simulink model "gm_quad_enc_fpga_pcie_slrt"  (R2020b)
settings: Solver=FixedStepDiscrete  StartTime=0.0  StopTime=5  FixedStep=1e-3  RelTol=1e-3
PostLoadFcn:
  | try
  | cell = struct2cell(dir(fullfile(speedgoatroot_hdlb, 'hdlsrc', 'quadrature', '*.vhd')));
  | addSourceFiles = strjoin(fullfile(cell(2,:),cell(1,:)), ';');
  | hdlset_param('quadrature_example_hdlc/DUT Quadrature', 'IPCoreAdditionalFiles', addSourceFiles);
  | end
undefined symbols (not defined in the file): IO334
libraries: speedgoatlib_hdlCoder_IO3xx x8, quadrature_cpulib x1
settings Model: ModifiedByFormat=Speedgoat GmbH  Creator=Speedgoat GmbH  LastModifiedBy=Speedgoat GmbH
settings SolverCC: ConcurrentTasks=on  PositivePriorityOrder=on
settings DataIOCC: ReturnWorkspaceOutputs=off
settings OptimizationCC: BlockReduction=off  ConditionallyExecuteInputs=off  DefaultParameterBehavior=Inlined  OptimizeBlockIOStorage=off
settings DebuggingCC: AlgebraicLoopMsg=error  TasksWithSamePriorityMsg=none  ParameterOverflowMsg=warning  PregeneratedLibrarySubsystemCodeDiagnostic=none  ArithmeticOperatorsInVariantConditions=warning
settings HardwareCC: ProdBitPerLong=64  ProdLongLongMode=on  ProdHWDeviceType=Intel->x86-64 (Linux 64)  TargetBitPerPointer=64  TargetBitPerSizeT=64  TargetBitPerPtrDiffT=64  TargetLongLongMode=on  TargetIntDivRoundTo=Zero  TargetEndianess=LittleEndian  TargetWordSize=64  TargetHWDeviceType=Custom Processor->MATLAB Host Computer
settings SFSimCC: SimUseLocalCustomCode=off  CustomCodeUndefinedFunction=UseInterfaceOnly
settings RTWCC: Description=Simulink Real-Time  SystemTargetFile=slrealtime.tlc  TemplateMakefile=slrealtime_default_tmf  RTWUseLocalCustomCode=off  Toolchain=Simulink Real-Time Toolchain  BuildConfiguration=Faster Runs  CodeExecutionProfiling=on  TargetLang=C++

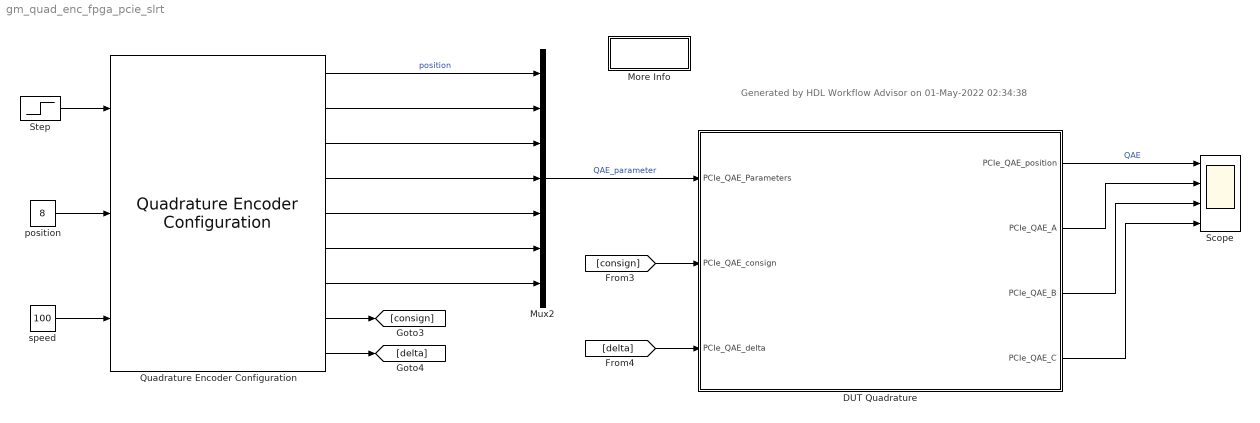
== system gm_quad_enc_fpga_pcie_slrt ==
  note: Generated by HDL Workflow Advisor on 01-May-2022 02:34:38
  DUT Quadrature : Subsystem  mask(Speedgoat IO334-325k Interface Block){module_id=1, slot=-1, ts=-1, FpgaFreq=100}
      mask prompts: module_id "FPGA Module Identifier:"; slot "PCI slot (-1: autosearch):"; ts "Sample time:"; FpgaFreq "FPGA Frequency [MHz]"
      mask help: Simulink Real-Time Interface Block for Speedgoat IO334-325k.
      mask init:
      | hdlslrt.backend.mfpgaparameters;
      mask Help: eval('speedgoatdoc_hdlc')
      mask Display:
      | SetupBlkPath = find_system(gcb, 'LookUnderMasks', 'all', 'FollowLinks', 'on', 'regexp', 'on', 'Name', 'IO3(\d|x){2}\s+Setup' );
      | SetupBlkPath = SetupBlkPath{1};
      | TS = get_param(SetupBlkPath,'timestamp_mcs');
      | disp(sprintf('Speedgoat IO334-325k\nFPGA I/O Module\n\nTimestamp\n%s\n\nReference Design\nVersion 2.1\n\nMatlab R2020b\n\nPCIe Link Width: X4\nRear Plugin: -21\nAurora Mode: None\nAurora Byteswap: true\n', TS))
  More Info : Subsystem
      settings: OpenFcn=|
      | try
      | speedgoat.hdlioblockset.doc('page', 'quadrature');
      | catch
      | web('https://www.speedgoat.com/help/hdlcoder/page/hdlb/refentry_hdl_blockset_quadrature');
      | end
      mask Display: disp('Documentation')
  Mux2 : Mux  Inputs=7
  Quadrature Encoder Configuration : quadrature_cpulib/Quadrature Encoder Configuration  fpgaFreq=100e6  n_channels=1  numSeg=[16]  phaseAngle=90  initPos=[0]  freeWheel=on
      settings: SourceProductName=Simulink Real-Time: Speedgoat HDL Blockset
  Scope : Scope  NumInputPorts=4
  Step : Step  Time=0.002
  position : Constant  Value=8  SampleTime=-1
  speed : Constant  Value=100  SampleTime=-1
  wires:
  Step/1 -> Quadrature Encoder Configuration/1
  DUT Quadrature/1(PCIe_QAE_position) -> Scope/1  "QAE"
  DUT Quadrature/4(PCIe_QAE_C) -> Scope/4
  DUT Quadrature/3(PCIe_QAE_B) -> Scope/3
  DUT Quadrature/2(PCIe_QAE_A) -> Scope/2
  Quadrature Encoder Configuration/5 -> Mux2/5
  [delta] -> DUT Quadrature/3(PCIe_QAE_delta)
  [consign] -> DUT Quadrature/2(PCIe_QAE_consign)
  Quadrature Encoder Configuration/4 -> Mux2/4
  Quadrature Encoder Configuration/1 -> Mux2/1  "position"
  Mux2/1 -> DUT Quadrature/1(PCIe_QAE_Parameters)  "QAE_parameter"
  Quadrature Encoder Configuration/9 -> [delta]
  Quadrature Encoder Configuration/8 -> [consign]
  Quadrature Encoder Configuration/7 -> Mux2/7
  Quadrature Encoder Configuration/6 -> Mux2/6
  Quadrature Encoder Configuration/3 -> Mux2/3
  Quadrature Encoder Configuration/2 -> Mux2/2
  speed/1 -> Quadrature Encoder Configuration/3
  position/1 -> Quadrature Encoder Configuration/2

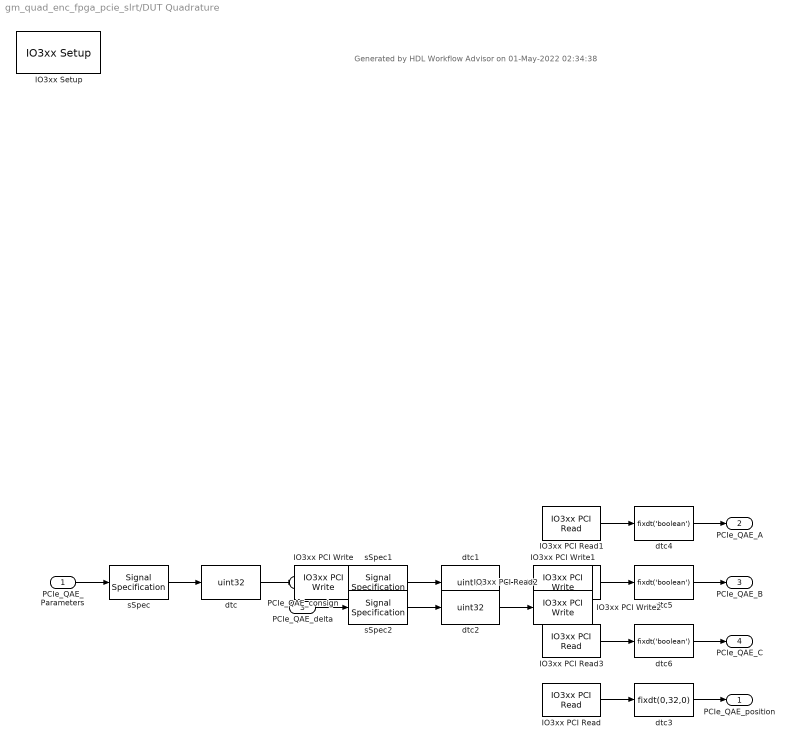
== system gm_quad_enc_fpga_pcie_slrt/DUT Quadrature ==
  note: Generated by HDL Workflow Advisor on 01-May-2022 02:34:38
  PCIe_QAE_Parameters : Inport
  PCIe_QAE_consign : Inport  Port=2  OutDataTypeStr=uint32  PortDimensions=1
  PCIe_QAE_delta : Inport  Port=3  PortDimensions=1
  IO3xx PCI Read : speedgoatlib_hdlCoder_IO3xx/IO3xx PCI Read  device_id=deviceIdx  module_id=module_id  board_type=IO3xx  port_name=PCIe_QAE_position  port_offset=hex2dec('130')  port_type=uint32  port_dim=1  strobe=0  sample_time=ts
  IO3xx PCI Read1 : speedgoatlib_hdlCoder_IO3xx/IO3xx PCI Read  device_id=deviceIdx  module_id=module_id  board_type=IO3xx  port_name=PCIe_QAE_A  port_offset=hex2dec('100')  port_type=uint32  port_dim=1  strobe=0  sample_time=ts
  IO3xx PCI Read2 : speedgoatlib_hdlCoder_IO3xx/IO3xx PCI Read  device_id=deviceIdx  module_id=module_id  board_type=IO3xx  port_name=PCIe_QAE_B  port_offset=hex2dec('104')  port_type=uint32  port_dim=1  strobe=0  sample_time=ts
  IO3xx PCI Read3 : speedgoatlib_hdlCoder_IO3xx/IO3xx PCI Read  device_id=deviceIdx  module_id=module_id  board_type=IO3xx  port_name=PCIe_QAE_C  port_offset=hex2dec('108')  port_type=uint32  port_dim=1  strobe=0  sample_time=ts
  IO3xx PCI Write : speedgoatlib_hdlCoder_IO3xx/IO3xx PCI Write  device_id=deviceIdx  module_id=module_id  board_type=IO3xx  port_name=PCIe_QAE_Parameters  port_offset=hex2dec('140')  port_type=uint32  port_dim=7  strobe=hex2dec('160')  sample_time=ts
  IO3xx PCI Write1 : speedgoatlib_hdlCoder_IO3xx/IO3xx PCI Write  device_id=deviceIdx  module_id=module_id  board_type=IO3xx  port_name=PCIe_QAE_consign  port_offset=hex2dec('128')  port_type=uint32  port_dim=1  strobe=0  sample_time=ts
  IO3xx PCI Write2 : speedgoatlib_hdlCoder_IO3xx/IO3xx PCI Write  device_id=deviceIdx  module_id=module_id  board_type=IO3xx  port_name=PCIe_QAE_delta  port_offset=hex2dec('12C')  port_type=uint32  port_dim=1  strobe=0  sample_time=ts
  IO3xx Setup : speedgoatlib_hdlCoder_IO3xx/IO3xx Setup  mdl_ss_name=quad_enc_fpga_pcie/DUT Quadrature  board_type=IO334-325k  fpga_sync_mode=on  reset_mode=on  device_id=deviceIdx  module_id=module_id  pci_slot=slot  fpga_mat_file=hdl_prj\hdlsrc\quad_enc_fpga_pcie\DUTQuadrature.mat  timestamp_mcs=05/01/22 02:23:06  timestamp=2205010147  tsreg=hex2dec('8')  bsf_file=DUTQuadrature_2205010147.mcs  mcs=0
  dtc : DataTypeConversion  OutDataTypeStr=uint32  ConvertRealWorld=Stored Integer (SI)  RndMeth=Zero
  dtc1 : DataTypeConversion  OutDataTypeStr=uint32  ConvertRealWorld=Stored Integer (SI)  RndMeth=Zero
  dtc2 : DataTypeConversion  OutDataTypeStr=uint32  ConvertRealWorld=Stored Integer (SI)  RndMeth=Zero
  dtc3 : DataTypeConversion  OutDataTypeStr=fixdt(0,32,0)  ConvertRealWorld=Stored Integer (SI)  RndMeth=Zero
  dtc4 : DataTypeConversion  OutDataTypeStr=fixdt('boolean')  ConvertRealWorld=Stored Integer (SI)  RndMeth=Zero
  dtc5 : DataTypeConversion  OutDataTypeStr=fixdt('boolean')  ConvertRealWorld=Stored Integer (SI)  RndMeth=Zero
  dtc6 : DataTypeConversion  OutDataTypeStr=fixdt('boolean')  ConvertRealWorld=Stored Integer (SI)  RndMeth=Zero
  sSpec : SignalSpecification  OutDataTypeStr=fixdt(0,32,0)
  sSpec1 : SignalSpecification  OutDataTypeStr=fixdt(0,32,0)
  sSpec2 : SignalSpecification  OutDataTypeStr=fixdt(1,32,0)
  PCIe_QAE_position : Outport  VectorParamsAs1DForOutWhenUnconnected=off
  PCIe_QAE_A : Outport  Port=2  VectorParamsAs1DForOutWhenUnconnected=off
  PCIe_QAE_B : Outport  Port=3  VectorParamsAs1DForOutWhenUnconnected=off
  PCIe_QAE_C : Outport  Port=4  VectorParamsAs1DForOutWhenUnconnected=off
  wires:
  PCIe_QAE_Parameters/1 -> sSpec/1
  sSpec/1 -> dtc/1
  dtc/1 -> IO3xx PCI Write/1
  PCIe_QAE_consign/1 -> sSpec1/1
  sSpec1/1 -> dtc1/1
  dtc1/1 -> IO3xx PCI Write1/1
  PCIe_QAE_delta/1 -> sSpec2/1
  sSpec2/1 -> dtc2/1
  dtc2/1 -> IO3xx PCI Write2/1
  dtc3/1 -> PCIe_QAE_position/1
  IO3xx PCI Read/1 -> dtc3/1
  dtc4/1 -> PCIe_QAE_A/1
  IO3xx PCI Read1/1 -> dtc4/1
  dtc5/1 -> PCIe_QAE_B/1
  IO3xx PCI Read2/1 -> dtc5/1
  dtc6/1 -> PCIe_QAE_C/1
  IO3xx PCI Read3/1 -> dtc6/1

== system gm_quad_enc_fpga_pcie_slrt/More Info ==
